simulink model "first1"  (R2014b)
settings: Solver=ode45  StartTime=0.0  StopTime=30  MaxStep=0.001  MinStep=0.0001  RelTol=1e-3
settings Model: Creator=Игорь  LastModifiedBy=Игорь

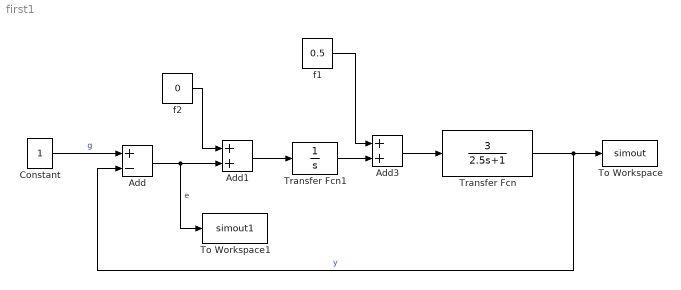
== system first1 ==
  Add : Sum  Inputs=+-
  Add1 : Sum
  Add3 : Sum
  Constant : Constant
  To Workspace : ToWorkspace  VariableName=simout  SaveFormat=Timeseries  SampleTime=-1
  To Workspace1 : ToWorkspace  VariableName=simout1  SaveFormat=Timeseries  SampleTime=-1
  Transfer Fcn : TransferFcn  Numerator=[3]  Denominator=[2.5 1]
  Transfer Fcn1 : TransferFcn  Denominator=[1 0]
  "f1 " : Constant  Value=0.5
  f2 : Constant  Value=0
  wires:
  Add/1 -> Add1/2, To Workspace1/1  "e"
  Constant/1 -> Add/1  "g"
  f2/1 -> Add1/1
  Transfer Fcn/1 -> Add/2, To Workspace/1  "y"
  Add1/1 -> Transfer Fcn1/1
  Transfer Fcn1/1 -> Add3/2
  Add3/1 -> Transfer Fcn/1
  "f1 "/1 -> Add3/1
